simulink model "mpc_soft_con"  (R2019b)
settings: Solver=VariableStepAuto  StartTime=0.0  StopTime=time_end  RelTol=1e-3
values from neighbouring files (symbols this model uses):
  h_01 = 10.17    [script_mpc_soft_con.m]
  h_02 = 10.53    [script_mpc_soft_con.m]
  Td = 0.5    [script_mpc_soft_con.m]
  u_max = repmat(u_max,Nc,1)    [script_mpc_soft_con.m]
  u_min = repmat(u_min,Nc,1)    [script_mpc_soft_con.m]
  ue = [ue1; ue2]    [script_mpc_soft_con.m]
  xe = [xe1; xe2]    [script_mpc_soft_con.m]
  xe1 = (k_2*sqrt(xe2)/k_1)^2    [script_mpc_soft_con.m]
  xe2 = 25.53    [script_mpc_soft_con.m]
undefined symbols (not defined in the file or in its folder): A, B, C, Fx, Fy, Gx, Gy
settings Model: Creator=NicSch02  LastModifiedBy=NicSch02

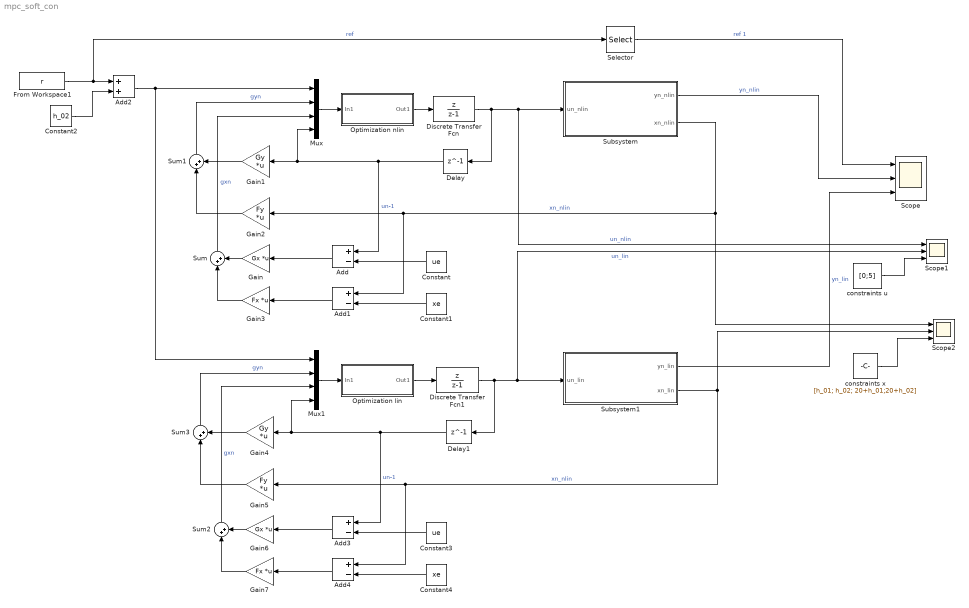
== system mpc_soft_con ==
  Add{,1,3..4} (4 alike) : Sum  Inputs=+-
  Add2 : Sum
  Constant : Constant  Value=ue
  Constant1 : Constant  Value=xe
  Constant2 : Constant  Value=h_02
  Constant3 : Constant  Value=ue
  Constant4 : Constant  Value=xe
  Delay : Delay  DelayLength=1  InitialCondition=[0;0]  SampleTime=Td
  Delay1 : Delay  DelayLength=1  InitialCondition=[0;0]  SampleTime=Td
  Discrete Transfer Fcn : DiscreteTransferFcn  Numerator=[1 0]  Denominator=[1 -1]  InitialStates=[0;0]  SampleTime=Td
  Discrete Transfer Fcn1 : DiscreteTransferFcn  Numerator=[1 0]  Denominator=[1 -1]  InitialStates=[0;0]  SampleTime=Td
  From Workspace1 : FromWorkspace  VariableName=r  SampleTime=0
  Gain : Gain  Gain=Gx  Multiplication=Matrix(K*u)
  Gain1 : Gain  Gain=Gy  Multiplication=Matrix(K*u)
  Gain2 : Gain  Gain=Fy  Multiplication=Matrix(K*u)
  Gain3 : Gain  Gain=Fx  Multiplication=Matrix(K*u)
  Gain4 : Gain  Gain=Gy  Multiplication=Matrix(K*u)
  Gain5 : Gain  Gain=Fy  Multiplication=Matrix(K*u)
  Gain6 : Gain  Gain=Gx  Multiplication=Matrix(K*u)
  Gain7 : Gain  Gain=Fx  Multiplication=Matrix(K*u)
  Mux : Mux
  Mux1 : Mux
  Optimization lin : Subsystem  TreatAsAtomicUnit=on  SystemSampleTime=Td
  Optimization nlin : Subsystem  TreatAsAtomicUnit=on  SystemSampleTime=Td
  Scope : Scope  NumInputPorts=3
  Scope1 : Scope  NumInputPorts=3
  Scope2 : Scope  NumInputPorts=3
  Selector : Selector  InputPortWidth=Np  IndexOptions=Index vector (dialog)  Indices=[1]  OutputSizes=1
  Subsystem : Subsystem
  Subsystem1 : Subsystem
  Sum{,1..3} (4 alike) : Sum  Inputs=|++
  constraints u : Constant  Value=[0;5]
  constraints x : Constant  Value=[h_01; h_02; 20+h_01;20+h_02]
  wires:
  Discrete Transfer Fcn/1 -> Scope1/1, Subsystem/1(un_nlin), Delay/1  "un_nlin"
  Delay/1 -> Add/1, Mux/4, Gain1/1  "un-1"
  Gain1/1 -> Sum1/2
  Sum1/1 -> Mux/2  "gyn"
  Gain2/1 -> Sum1/1
  Subsystem/1(yn_nlin) -> Scope/2  "yn_nlin"
  Discrete Transfer Fcn1/1 -> Scope1/2, Subsystem1/1(un_lin), Delay1/1  "un_lin"
  Gain4/1 -> Sum3/2
  Gain5/1 -> Sum3/1
  Subsystem1/1(yn_lin) -> Scope/3  "yn_lin"
  Subsystem/2(xn_nlin) -> Add1/1, Gain2/1, Scope2/1  "xn_nlin"
  Selector/1 -> Scope/1  "ref 1"
  Mux/1 -> Optimization nlin/1(In1)
  Sum3/1 -> Mux1/2  "gyn"
  Mux1/1 -> Optimization lin/1(In1)
  Optimization nlin/1(Out1) -> Discrete Transfer Fcn/1
  Optimization lin/1(Out1) -> Discrete Transfer Fcn1/1
  Gain/1 -> Sum/2
  Gain3/1 -> Sum/1
  Sum/1 -> Mux/3  "gxn"
  Gain6/1 -> Sum2/2
  Sum2/1 -> Mux1/3  "gxn"
  Gain7/1 -> Sum2/1
  Constant2/1 -> Add2/2
  From Workspace1/1 -> Selector/1, Add2/1  "ref"
  Add2/1 -> Mux1/1, Mux/1
  constraints x/1 -> Scope2/3
  constraints u/1 -> Scope1/3
  Add/1 -> Gain/1
  Add1/1 -> Gain3/1
  Constant/1 -> Add/2
  Constant1/1 -> Add1/2
  Add4/1 -> Gain7/1
  Constant3/1 -> Add3/2
  Add3/1 -> Gain6/1
  Subsystem1/2(xn_lin) -> Add4/1, Gain5/1, Scope2/2  "xn_nlin"
  Constant4/1 -> Add4/2
  Delay1/1 -> Add3/1, Mux1/4, Gain4/1  "un-1"

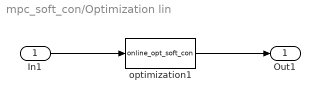
== system mpc_soft_con/Optimization lin ==
  In1 : Inport
  optimization1 : MATLABFcn  MATLABFcn=online_opt_soft_con
  Out1 : Outport
  wires:
  In1/1 -> optimization1/1
  optimization1/1 -> Out1/1

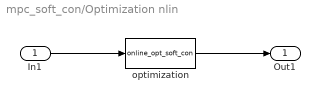
== system mpc_soft_con/Optimization nlin ==
  In1 : Inport
  optimization : MATLABFcn  MATLABFcn=online_opt_soft_con
  Out1 : Outport
  wires:
  In1/1 -> optimization/1
  optimization/1 -> Out1/1

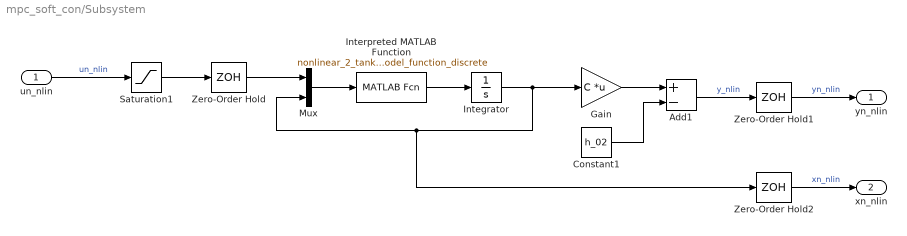
== system mpc_soft_con/Subsystem ==
  un_nlin : Inport
  Add1 : Sum  Inputs=+-
  Constant1 : Constant  Value=h_02
  Gain : Gain  Gain=C  Multiplication=Matrix(K*u)
  Integrator : Integrator  InitialCondition=[h_01;h_02]
  Interpreted MATLAB Function : MATLABFcn  MATLABFcn=nonlinear_2_tank_model_function_discrete
  Mux : Mux  Inputs=2
  Saturation1 : Saturate  UpperLimit=u_max(1)  LowerLimit=u_min(1)
  Zero-Order Hold : ZeroOrderHold  SampleTime=Td
  Zero-Order Hold1 : ZeroOrderHold  SampleTime=Td
  Zero-Order Hold2 : ZeroOrderHold  SampleTime=Td
  yn_nlin : Outport
  xn_nlin : Outport  Port=2
  wires:
  Integrator/1 -> Zero-Order Hold2/1, Mux/2, Gain/1
  Constant1/1 -> Add1/2
  Interpreted MATLAB Function/1 -> Integrator/1
  Gain/1 -> Add1/1
  Mux/1 -> Interpreted MATLAB Function/1
  un_nlin/1 -> Saturation1/1  "un_nlin"
  Zero-Order Hold/1 -> Mux/1
  Add1/1 -> Zero-Order Hold1/1  "y_nlin"
  Zero-Order Hold1/1 -> yn_nlin/1  "yn_nlin"
  Saturation1/1 -> Zero-Order Hold/1
  Zero-Order Hold2/1 -> xn_nlin/1  "xn_nlin"

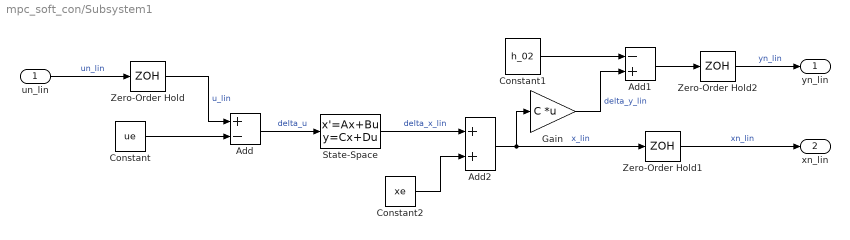
== system mpc_soft_con/Subsystem1 ==
  un_lin : Inport
  Add : Sum  Inputs=+-
  Add1 : Sum  Inputs=-+
  Add2 : Sum
  Constant : Constant  Value=ue
  Constant1 : Constant  Value=h_02
  Constant2 : Constant  Value=xe
  Gain : Gain  Gain=C  Multiplication=Matrix(K*u)
  State-Space : StateSpace  A=A  B=B  C=[[1,0];[0,1]]  D=[[0,0];[0,0]]  InitialCondition=[h_01;h_02] - [xe1; xe2]
  Zero-Order Hold : ZeroOrderHold  SampleTime=Td
  Zero-Order Hold1 : ZeroOrderHold  SampleTime=Td
  Zero-Order Hold2 : ZeroOrderHold  SampleTime=Td
  yn_lin : Outport
  xn_lin : Outport  Port=2
  wires:
  Constant/1 -> Add/2
  Add/1 -> State-Space/1  "delta_u"
  Constant2/1 -> Add2/2
  State-Space/1 -> Add2/1  "delta_x_lin"
  un_lin/1 -> Zero-Order Hold/1  "un_lin"
  Zero-Order Hold/1 -> Add/1  "u_lin"
  Add2/1 -> Zero-Order Hold1/1, Gain/1  "x_lin"
  Zero-Order Hold1/1 -> xn_lin/1  "xn_lin"
  Zero-Order Hold2/1 -> yn_lin/1  "yn_lin"
  Add1/1 -> Zero-Order Hold2/1
  Constant1/1 -> Add1/1
  Gain/1 -> Add1/2  "delta_y_lin"
